simulink model "Battery_50kw_AC_500KW_400V_pruebas_2020_2_individual"  (R2020b)
settings: Solver=VariableStepAuto  StartTime=0.0  StopTime=0.4  RelTol=1e-3
InitFcn:
  | Ts=100e-6;
  | Timer=0.001;
StartFcn:
  | Ts=100e-6;
  | Timer=0.001;
undefined symbols (not defined in the file or in its folder): Ion, Lithium
libraries: powerlib x44, powerlib_meascontrol x16, slpidlib x10, simulink x5, electricdrivelib x1
(part 1 of 2)
settings Model: Creator=JGC  LastModifiedBy=DGY
settings DataIOCC: ReturnWorkspaceOutputs=off

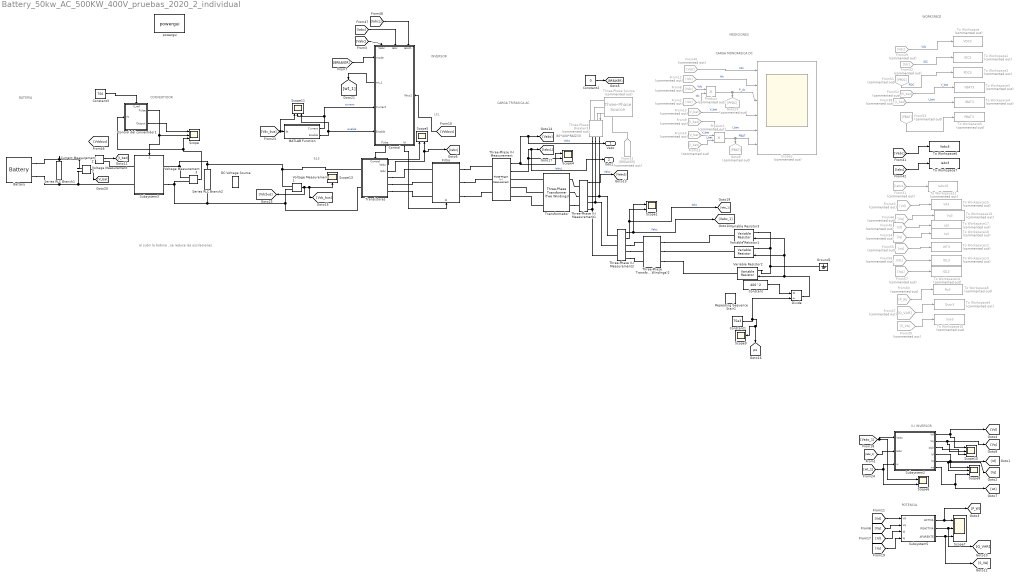
== system Battery_50kw_AC_500KW_400V_pruebas_2020_2_individual ==
  note: al subir la bobina , se reduce las oscilaciones
  note: WORKSPACE
  note: CARGA MONOFASICA DC
  note: MEDICIONES
  note: CONVERTIDOR
  note: INVERSOR
  note: BATERIA
  note: 80*400*RAIZ(3)
  note: CARGA TRIFASICA AC
  note: 615
  note: LCL
  note: V-I INVERSOR
  note: POTENCIA
  Battery : electricdrivelib/Extra Sources/Battery  BatType=Lithium-Ion  ShowTempParam=off  ThermalPreset=no  ShowAgeParam=off  NomV=512  NomQ=102400/512  SOC=70  Batt_Tr=30  PresetModel=on  MaxQ=200  MinV=384  FullV=595.9614  Dis_rate=86.9565  R=0.0256  Normal_OP=180.8696  expZone="[553.1576      9.826087]"  current=[6.5 13 32.5]  Units=Time  Tci=20  NomT=20  T2=-30  MaxQ2=4.8  FullV2=7.1  Normal_OP2=5.655  expZone2="[6.58           1]"  Rca=0.6  ti=2000  Dp=0  Neq0=0  Tsim=1e6  Ta1=25  Qeol=5.4*0.9  Reol=0.013333*1.2  Char_age=[2.3478, 3]  Dis_age=[2.3478, 10]  N1=1500  N2=10500  N3=1000  N4=1400  Ta2=45  N5=950
  Constant : Constant  Value=400^2
  Constant1 : Constant  Value=75e3
  Constant2 : Constant  Value=0
  Constant3 : Constant  Value=750
  "Control " : Subsystem
      settings: PortSchema="{\"entries\":[{\"content\":{\"sides\":[{\"content\":{\"connectorIds\":[\"In1\",\"Out3\",\"In2\",\"In3\"]},\"type\":\"ConnectorPlacement.EquallySpacedRectSide\",\"uuid\":\"040f479b-0063-4a97-945a-b7b76c14ccf9\"},{\"content\":{\"connectorIds\":[\"In7\"],\"side\":\"RIGHT\"},\"type\":\"ConnectorPlacement.EquallySpacedRectSide\",\"uuid\":\"48d15187-e0ba-47e4-acd1-e370322fb20d\"},{\"content\":{\"connectorIds\":[\"In4\",\"In5\",\"In6\"],\"side\":\"TOP\"},\"type\":\"ConnectorPlacement.EquallySpacedRectSide\",\"uuid\":\"c47ff363-741e-4c95-9660-92ffbbf0858a\"},{\"content\":{\"connectorIds\":[\"Out1\",\"Out2\"],\"side\":\"BOTTOM\"},\"type\":\"ConnectorPlacement.EquallySpacedRectSide\",\"uuid\":\"eb550659-5dfa-48af-9c5b-3062ad81491f\"}]},\"type\":\"ConnectorPlacement.EquallySpacedConnector\",\"uuid\":\"b4b94fd9-d3fa-4033-a0eb-720d35d74a7d\"}],\"packageUris\":[\"http://schema.mathworks.com/mf0/Connector/R2020b\"],\"version\":\"1.0\"}"
  Control del convertidor1 : Subsystem
      settings: PortSchema="{\"entries\":[{\"content\":{\"sides\":[{\"content\":{\"connectorIds\":[\"In1\"]},\"type\":\"ConnectorPlacement.EquallySpacedRectSide\",\"uuid\":\"952f4d9f-85a3-4809-ab80-f95b4e630059\"},{\"content\":{\"connectorIds\":[\"Out1\",\"Out2\"],\"side\":\"RIGHT\"},\"type\":\"ConnectorPlacement.EquallySpacedRectSide\",\"uuid\":\"24c0a236-3f22-4c40-86cc-925551a19bc9\"},{\"content\":{\"connectorIds\":[\"In2\"],\"side\":\"TOP\"},\"type\":\"ConnectorPlacement.EquallySpacedRectSide\",\"uuid\":\"1a366aec-943f-41ae-ba47-6c948c084703\"}]},\"type\":\"ConnectorPlacement.EquallySpacedConnector\",\"uuid\":\"c6d9e875-0dde-4ffd-9bd0-64114f723d5e\"}],\"packageUris\":[\"http://schema.mathworks.com/mf0/Connector/R2020b\"],\"version\":\"1.0\"}"
  Current Measurement2 : powerlib/Measurements/Current Measurement  PhasorSimulation=off  OutputType=Complex  PSBequivalent=0
  DC Voltage Source : powerlib/Electrical Sources/DC Voltage Source  Amplitude=750  Measurements=None
  Divide : Product  Inputs=*/
  Filtro : Subsystem
      settings: PortSchema="{\"entries\":[{\"content\":{\"sides\":[{\"content\":{\"connectorIds\":[\"LConn1\",\"LConn2\",\"LConn3\"]},\"type\":\"ConnectorPlacement.EquallySpacedRectSide\",\"uuid\":\"44f292cd-7929-4e59-9d40-ef793941fadf\"},{\"content\":{\"connectorIds\":[\"RConn1\",\"RConn2\",\"RConn3\"],\"side\":\"RIGHT\"},\"type\":\"ConnectorPlacement.EquallySpacedRectSide\",\"uuid\":\"e88b12c4-b753-4f44-a76b-0d232ef629de\"},{\"content\":{\"side\":\"TOP\"},\"type\":\"ConnectorPlacement.EquallySpacedRectSide\",\"uuid\":\"3a4dfe0a-8373-429f-aa79-480f87b68f50\"},{\"content\":{\"connectorIds\":[\"In1\"],\"side\":\"BOTTOM\"},\"type\":\"ConnectorPlacement.EquallySpacedRectSide\",\"uuid\":\"d1028483-6dfb-4af9-bac2-a2f24ebe33e6\"}]},\"type\":\"ConnectorPlacement.EquallySpacedConnector\",\"uuid\":\"17b3d09e-bad1-4b7f-8a8e-7737b1d04969\"}],\"packageUris\":[\"http://schema.mathworks.com/mf0/Connector/R2020b\"],\"version\":\"1.0\"}"
  From12 : From  Commented=on  GotoTag=Idc
  From13 : From  Commented=on  GotoTag=V_bat
  From14 : From  Commented=on  GotoTag=V_bat
  From15 : From  Commented=on  GotoTag=I_bat
  From2 : From  Commented=on  GotoTag=Idc
  From29 : From  Commented=on  GotoTag=Vdc
  From30 : From  Commented=on  GotoTag=P_W
  From31 : From  Commented=on  GotoTag=IabcL
  From32 : From  Commented=on  GotoTag=Idc
  From33 : From  Commented=on  GotoTag=BREAKER
  From37 : From  Commented=on  GotoTag=Q_VAR
  From38 : From  Commented=on  GotoTag=I_bat
  From39 : From  Commented=on  GotoTag=S_VA
  From40 : From  Commented=on  GotoTag=Vdc
  From43 : From  Commented=on  GotoTag=Vd
  From44 : From  Commented=on  GotoTag=Vq
  From45 : From  Commented=on  GotoTag=Id
  From51 : From  Commented=on  GotoTag=PPDC
  From52 : From  Commented=on  GotoTag=V_bat
  From53 : From  Commented=on  GotoTag=PBAT
  From54 : From  Commented=on  GotoTag=Iq
  From55 : From  Commented=on  GotoTag=wt
  From56 : From  Commented=on  GotoTag=IdL
  From57 : From  Commented=on  GotoTag=IqL
  From8 : From  Commented=on  GotoTag=Vdc
  From9 : From  Commented=on  GotoTag=I_bat
  Goto23 : Goto  Commented=on  GotoTag=PPDC
  Goto9 : Goto  Commented=on  GotoTag=PBAT
  Ground1 : powerlib/Elements/Ground  LConnTagsString=a
  MATLAB Function : MATLAB Function  TreatAsAtomicUnit=on
  Product : Product  Commented=on
  Product1 : Product  Commented=on
  Repeating Sequence Stair1 : simulink/Sources/Repeating Sequence Stair  OutValues=[ 30e3 35e3 45e3 50e3 40e3].'  tsamp=0.08  OutMin=[]  OutMax=[]  OutDataTypeStr=double  OutputDataTypeScalingMode=double  OutDataType=fixdt(0,8)  ConRadixGroup=Best Precision: Vector-wise  OutScaling=2^-12
  Scope{,7..8,10..11} (5 alike) : Scope  NumInputPorts=3
  Scope{1,4..6} (4 alike) : Scope  NumInputPorts=2
  Scope13 : Scope
  Scope2 : Scope  Commented=on  NumInputPorts=6
  Scope9 : Scope
  Series RLC Branch1 : powerlib/Elements/Series RLC Branch  LConnTagsString=__new0  RConnTagsString=__new0  BranchType=RC  Resistance=0.3  Inductance=1e-3  SetiL0=off  InitialCurrent=0  Capacitance=1e-6  Setx0=on  InitialVoltage=512  Measurements=None
  Series RLC Branch2 : powerlib/Elements/Series RLC Branch  LConnTagsString=__new0  RConnTagsString=__new0  BranchType=C  Resistance=0.2  Inductance=1e-3  SetiL0=off  InitialCurrent=0  Capacitance=0.15  Setx0=on  InitialVoltage=600  Measurements=None
  Subsystem2 : Subsystem
  Subsystem3 : Subsystem
      settings: PortSchema="{\"entries\":[{\"content\":{\"sides\":[{\"content\":{\"connectorIds\":[\"LConn1\",\"LConn2\"]},\"type\":\"ConnectorPlacement.EquallySpacedRectSide\",\"uuid\":\"7a980847-0fd3-4a52-ae22-59cd2a1ed559\"},{\"content\":{\"connectorIds\":[\"RConn1\",\"RConn2\"],\"side\":\"RIGHT\"},\"type\":\"ConnectorPlacement.EquallySpacedRectSide\",\"uuid\":\"85effeeb-73a6-4b0a-b51b-5eb0082317ff\"},{\"content\":{\"connectorIds\":[\"In1\"],\"side\":\"TOP\"},\"type\":\"ConnectorPlacement.EquallySpacedRectSide\",\"uuid\":\"eb55fae0-79ad-414f-ab96-49c332138803\"},{\"content\":{\"side\":\"BOTTOM\"},\"type\":\"ConnectorPlacement.EquallySpacedRectSide\",\"uuid\":\"1fd972ff-419a-4657-8ea4-57d89be2b868\"}]},\"type\":\"ConnectorPlacement.EquallySpacedConnector\",\"uuid\":\"1807473d-fd42-44e0-a7e4-668a7bf21429\"}],\"packageUris\":[\"http://schema.mathworks.com/mf0/Connector/R2020b\"],\"version\":\"1.0\"}"
  Subsystem5 : Subsystem
  Three-Phase Transformer (Two Windings)2 : powerlib/Elements/Three-Phase Transformer (Two Windings)  Winding1Connection=Yg  Winding2Connection=Yg  CoreType=Three single-phase transformers  SetSaturation=off  Hysteresis=off  DataFile='hysteresis'  SetInitialFlux=off  Measurements=None  UNITS=SI  NominalPower=[ 50e3 , 50 ]  Winding1=[400 0.0064 0]  Winding2=[400 0.0064 0]  Rm=1600  Lm=0  L0=0.5  Saturation=[0 0;0.24495 1.2475;102.06 1.5802]  InitialFluxes=[ 0.8 , -0.8 , 0.7 ]  BreakLoop=off  DiscreteSolver=Trapezoidal iterative  DataType=on  TransfoNumber=1
  Three-Phase V-I Measurement : powerlib/Measurements/Three-Phase V-I Measurement  VoltageMeasurement=phase-to-phase  SetLabelV=off  LabelV=Vabc  Vpu=off  VpuLL=off  CurrentMeasurement=yes  SetLabelI=off  LabelI=Iabc  Ipu=off  Pbase=100e6  Vbase=500e3  OutputType=Complex  PhasorSimulation=off  PSBequivalent=0
  Three-Phase V-I Measurement1 : powerlib/Measurements/Three-Phase V-I Measurement  VoltageMeasurement=phase-to-phase  SetLabelV=off  LabelV=Vabc  Vpu=off  VpuLL=off  CurrentMeasurement=yes  SetLabelI=off  LabelI=Iabc  Ipu=off  Pbase=100e6  Vbase=500e3  OutputType=Complex  PhasorSimulation=off  PSBequivalent=0
  Three-Phase V-I Measurement2 : powerlib/Measurements/Three-Phase V-I Measurement  VoltageMeasurement=phase-to-phase  SetLabelV=off  LabelV=Vabc  Vpu=off  VpuLL=off  CurrentMeasurement=yes  SetLabelI=off  LabelI=Iabc  Ipu=off  Pbase=100e6  Vbase=500e3  OutputType=Complex  PhasorSimulation=off  PSBequivalent=0
  Three-Phase Breaker3 : powerlib/Elements/Three-Phase Breaker  Commented=on  InitialState=closed  SwitchA=on  SwitchB=on  SwitchC=on  SwitchTimes="[1/60  5/60]"  External=on  BreakerResistance=0.01  SnubberResistance=1e6  SnubberCapacitance=inf  Measurements=None
  Three-Phase Source : powerlib/Electrical Sources/Three-Phase Source  Commented=on  InternalConnection=Y  VoltagePhases=off  Voltage=400  PhaseAngle=0  Voltage_phases=[25e3 25e3 25e3]/sqrt(3)  PhaseAngles_phases=[0 -120 +120]  Frequency=50  NonIdealSource=on  SpecifyImpedance=off  Resistance=0.0001e-3  Inductance=0.0001e-9  ShortCircuitLevel=100e6  BaseVoltage=400  XRratio=7  BusType=swing  Pref=10e3  Qref=0  Prefabc=[10e3, 10e3, 10e3]  Qrefabc=[0, 0, 0]  Qmin=-inf  Qmax=inf
  To Workspace : ToWorkspace  Commented=on  VariableName=VDC3  SaveFormat=Timeseries  SampleTime=-1
  To Workspace1 : ToWorkspace  Commented=on  VariableName=IDC3  SaveFormat=Timeseries  SampleTime=-1
  To Workspace10 : ToWorkspace  Commented=on  VariableName=Sva3  SaveFormat=Timeseries  SampleTime=-1
  To Workspace11 : ToWorkspace  Commented=on  VariableName=IabcL5  SaveFormat=Structure With Time  SampleTime=-1
  To Workspace12 : ToWorkspace  Commented=on  VariableName=WT3  SaveFormat=Timeseries  SampleTime=-1
  To Workspace13 : ToWorkspace  Commented=on  VariableName=IDL3  SaveFormat=Timeseries  SampleTime=-1
  To Workspace14 : ToWorkspace  Commented=on  VariableName=IQL3  SaveFormat=Timeseries  SampleTime=-1
  To Workspace15 : ToWorkspace  Commented=on  VariableName=Vd3  SaveFormat=Timeseries  SampleTime=-1
  To Workspace16 : ToWorkspace  Commented=on  VariableName=Vq3  SaveFormat=Timeseries  SampleTime=-1
  To Workspace17 : ToWorkspace  Commented=on  VariableName=Id3  SaveFormat=Timeseries  SampleTime=-1
  To Workspace18 : ToWorkspace  Commented=on  VariableName=Iq3  SaveFormat=Timeseries  SampleTime=-1
  To Workspace2 : ToWorkspace  Commented=on  VariableName=PDC3  SaveFormat=Timeseries  SampleTime=-1
  To Workspace3 : ToWorkspace  Commented=on  VariableName=VBAT3  SaveFormat=Timeseries  SampleTime=-1
  To Workspace4 : ToWorkspace  Commented=on  VariableName=IBAT3  SaveFormat=Timeseries  SampleTime=-1
  To Workspace5 : ToWorkspace  Commented=on  VariableName=PBAT3  SaveFormat=Timeseries  SampleTime=-1
  To Workspace6 : ToWorkspace  VariableName=Vabc5  SaveFormat=Structure With Time  SampleTime=-1
  To Workspace7 : ToWorkspace  VariableName=Iabc3  SaveFormat=Timeseries  SampleTime=-1
  To Workspace8 : ToWorkspace  Commented=on  VariableName=Pw3  SaveFormat=Timeseries  SampleTime=-1
  To Workspace9 : ToWorkspace  Commented=on  VariableName=Qvar3  SaveFormat=Timeseries  SampleTime=-1
  "Transformador " : powerlib/Elements/Three-Phase Transformer (Two Windings)  Winding1Connection=Yg  Winding2Connection=Yg  CoreType=Three single-phase transformers  SetSaturation=off  Hysteresis=off  DataFile='hysteresis'  SetInitialFlux=off  Measurements=None  UNITS=SI  NominalPower=[50e3 , 50 ]  Winding1=[400 0.0064 0]  Winding2=[400 0.0064 0]  Rm=1600  Lm=0  L0=0.5  Saturation=[0 0;0.24495 1.2475;102.06 1.5802]  InitialFluxes=[ 0.8 , -0.8 , 0.7 ]  BreakLoop=off  DiscreteSolver=Trapezoidal iterative  DataType=on  TransfoNumber=1
  Transistores : Subsystem
      settings: PortSchema="{\"entries\":[{\"content\":{\"sides\":[{\"content\":{\"connectorIds\":[\"LConn1\",\"LConn2\"]},\"type\":\"ConnectorPlacement.EquallySpacedRectSide\",\"uuid\":\"4b4a90af-a54c-4879-a767-640ef5f3fcb3\"},{\"content\":{\"connectorIds\":[\"Out1\",\"Out2\",\"RConn1\",\"RConn2\",\"RConn3\"],\"side\":\"RIGHT\"},\"type\":\"ConnectorPlacement.EquallySpacedRectSide\",\"uuid\":\"9175716d-9f9b-4229-800b-ed18d0bc4919\"},{\"content\":{\"connectorIds\":[\"In1\"],\"side\":\"TOP\"},\"type\":\"ConnectorPlacement.EquallySpacedRectSide\",\"uuid\":\"ad8bb3e4-0cf0-4c72-aeb3-553776322e14\"}]},\"type\":\"ConnectorPlacement.EquallySpacedConnector\",\"uuid\":\"7a2ee168-b262-4afb-be64-1e845efa873f\"}],\"packageUris\":[\"http://schema.mathworks.com/mf0/Connector/R2020b\"],\"version\":\"1.0\"}"
  Variable Resistor1 : powerlib/Elements/Variable Resistor  Rabsmin=1e-3
      settings: SourceProductBaseCode=PS
  Variable Resistor2 : powerlib/Elements/Variable Resistor  Rabsmin=1e-3
      settings: SourceProductBaseCode=PS
  Variable Resistor3 : powerlib/Elements/Variable Resistor  Rabsmin=1e-3
      settings: SourceProductBaseCode=PS
  Voltage Measurement1 : powerlib/Measurements/Voltage Measurement  PhasorSimulation=off  OutputType=Complex  PSBequivalent=0
  Voltage Measurement2 : powerlib/Measurements/Voltage Measurement  PhasorSimulation=off  OutputType=Complex  PSBequivalent=0
  Voltage Measurement3 : powerlib/Measurements/Voltage Measurement  PhasorSimulation=off  OutputType=Complex  PSBequivalent=0
  powergui : powerlib/powergui  Priority=1  SimulationMode=Discrete  SampleTime=1e-5*3  frequency=60  Iterations=50  frequencyindice=0  Pbase=100e6  ErrMax=1e-4  UnitsV=kV  UnitsW=MW  buscounter=0  FunctionMessages=off  echomessages=off  EnableUseOfTLC=off  CurrentSourceSwitches=off  DisableSnubberDevices=off  DisableRonSwitches=off  DisableVfSwitches=off  DisplayEquations=off  AutomaticDiscreteSolvers=off  SolverType=Tustin/Backward Euler (TBE)  Interpol=off  ExternalGateDelay=off  methode=off  Ts=100  x0status=blocks  SPID=on  SwTol=0  HookPort=off  NonlinearTolerance=1e-4  nMaxIteration=100  ContinueOnMaxIteration=off  RestoreLinks=warning  ResistiveCurrentMeasurement=off  Frange=[0:2:500]  Ylog=off  Xlog=on  ShowGrid=off  save=off  variable=ZData  structure=IDC  ZoomFFT=off  StartTime=0.01  cycles=7  DisplayStyle=1  fundamental=50  FreqAxis=off  MaxFrequency=10000  frequencyindicesteady=1  RmsSteady=1  display=off
  Vabc : Outport
  IabcL : Outport  Port=2
  tag scope: po=global
  wires:
  MATLAB Function/1(Current) -> Scope11/2, "Control "/2(Current)  "current"
  [BREAKER] -> "Control "/1(mode)
  From32/1 -> To Workspace1/1  "IDC"
  From30/1 -> To Workspace8/1
  From38/1 -> To Workspace4/1  "I_bat"
  From29/1 -> To Workspace/1  "Vdc"
  From45/1 -> To Workspace17/1
  [Vdc_bus] -> MATLAB Function/1(IN), Scope11/1
  From37/1 -> To Workspace9/1
  Transistores/1(Vabc) -> Scope5/1
  [Vdcbus] -> "Control "/7(Vbus1)
  From57/1 -> To Workspace14/1
  From51/1 -> To Workspace2/1  "PDC"
  From2/1 -> Product/2  "Idc"
  [Iabc] -> To Workspace7/1
  From52/1 -> To Workspace3/1  "V_bat"
  From39/1 -> To Workspace10/1
  From53/1 -> To Workspace5/1
  From54/1 -> To Workspace18/1
  From56/1 -> To Workspace13/1
  From40/1 -> Scope2/1  "Vdc"
  From44/1 -> To Workspace16/1
  Transistores/2(Iabc) -> Scope5/2, [Iabc]
  Product1/1 -> Goto9/1, Scope2/6  "PBAT"
  From9/1 -> Scope2/5  "I_bat"
  Product/1 -> Goto23/1, Scope2/3  "P_dc"
  From8/1 -> Product/1  "Vdc"
  From13/1 -> Scope2/4  "V_bat"
  From14/1 -> Product1/1  "V_bat"
  From12/1 -> Scope2/2  "Idc"
  "Control "/1(Pulse) -> Transistores/1(Control)
  From15/1 -> Product1/2  "I_bat"
  From31/1 -> To Workspace11/1
  [Vabc] -> To Workspace6/1
  From55/1 -> To Workspace12/1
  Three-Phase V-I Measurement/1 -> Scope4/1, [Vabc], Vabc/1  "Vabc"
  From43/1 -> To Workspace15/1
  Three-Phase V-I Measurement/2 -> Scope4/2, [IabcL], IabcL/1  "IabcL"
  MATLAB Function/2(Enable) -> Scope11/3, "Control "/3(Enable)  "enable"
  Divide/1 -> Variable Resistor2/1, Variable Resistor3/1, Variable Resistor1/1
  Constant/1 -> Divide/1
  Three-Phase V-I Measurement1/1 -> [VabcS]  "Vabc"
  Constant2/1 -> [BREAKER]
  From33/1 -> Three-Phase Breaker3/1
  Voltage Measurement1/1 -> [Vdcbus], Scope13/1, [Vdc_bus]
  "Control "/2(Id) -> Filtro/1(Id)
  Control del convertidor1/1(Pulse) -> Subsystem3/1(S), Scope/2
  Voltage Measurement2/1 -> [V_bat]
  Current Measurement2/1 -> [I_bat]
  Voltage Measurement3/1 -> Control del convertidor1/1(Vs), Scope/3
  Constant3/1 -> Control del convertidor1/2(V_ref)
  Control del convertidor1/2(Output) -> Scope/1
  Constant1/1 -> Divide/2, Scope9/1, [po]
  [Vabc] -> "Control "/4(Vabc)
  [Iabc] -> "Control "/5(Iabc)
  [IabcL] -> "Control "/6(Iabcl1)
  Three-Phase V-I Measurement2/1 -> [Vabc_1], Scope1/1  "Vabc"
  Three-Phase V-I Measurement2/2 -> [Iabc_1], Scope1/2  "Iabc"
  Subsystem2/2(Vq) -> Scope10/2, [Vq]
  [Id] -> Subsystem5/3(Id)
  Subsystem5/1(ACTIVA) -> [P_W], Scope7/1
  Subsystem2/1(Vd) -> Scope10/1, [Vd]
  [Iq] -> Subsystem5/4(Iq)
  [Vabc_1] -> Scope6/1, Subsystem2/1(Vabc)
  Subsystem5/3(APARENTE) -> [S_VA], Scope7/3
  [Vd] -> Subsystem5/1(Vd)
  [Iabc_1] -> Subsystem2/2(Iabc)
  [Vq] -> Subsystem5/2(Vq)
  Subsystem2/3(dq0) -> Scope10/3
  [wt_1] -> Subsystem2/3(w), Scope6/2
  Subsystem2/6(wt) -> [wt], Scope8/3
  Subsystem2/4(Id) -> [Id], Scope8/1
  Subsystem5/2(REACTIVA) -> [Q_VAR], Scope7/2
  Subsystem2/5(Iq) -> Scope8/2, [Iq]
  "Control "/3(wt_1) -> [wt_1]
  connections:
  Filtro/LConn3 -- Three-Phase V-I Measurement/LConn3
  Transistores/RConn1 -- Filtro/RConn1
  Transistores/RConn2 -- Filtro/RConn2
  Filtro/LConn1 -- Three-Phase V-I Measurement/LConn1
  Filtro/LConn2 -- Three-Phase V-I Measurement/LConn2
  Transistores/RConn3 -- Filtro/RConn3
  Variable Resistor3/LConn1 -- Variable Resistor1/LConn1 -- Variable Resistor2/LConn1 -- Ground1/LConn1
  Three-Phase V-I Measurement1/RConn1 -- Three-Phase Breaker3/RConn1 -- Three-Phase V-I Measurement2/LConn1
  Three-Phase V-I Measurement1/RConn2 -- Three-Phase Breaker3/RConn2 -- Three-Phase V-I Measurement2/LConn2
  Three-Phase V-I Measurement1/RConn3 -- Three-Phase Breaker3/RConn3 -- Three-Phase V-I Measurement2/LConn3
  "Transformador "/LConn2 -- Three-Phase V-I Measurement/RConn2
  "Transformador "/LConn3 -- Three-Phase V-I Measurement/RConn3
  Three-Phase V-I Measurement1/LConn1 -- "Transformador "/RConn1
  "Transformador "/RConn2 -- Three-Phase V-I Measurement1/LConn2
  "Transformador "/LConn1 -- Three-Phase V-I Measurement/RConn1
  "Transformador "/RConn3 -- Three-Phase V-I Measurement1/LConn3
  Three-Phase Source/RConn2 -- Three-Phase Breaker3/LConn2
  Three-Phase Source/RConn1 -- Three-Phase Breaker3/LConn1
  Three-Phase Source/RConn3 -- Three-Phase Breaker3/LConn3
  Series RLC Branch1/LConn1 -- Battery/LConn1 -- Voltage Measurement2/LConn1 -- Current Measurement2/LConn1
  Series RLC Branch1/RConn1 -- Battery/LConn2 -- Voltage Measurement2/LConn2 -- Subsystem3/LConn2
  Subsystem3/LConn1 -- Current Measurement2/RConn1
  Subsystem3/RConn2 -- Voltage Measurement3/LConn2 -- Transistores/LConn2 -- Voltage Measurement1/LConn2 -- Series RLC Branch2/RConn1
  Subsystem3/RConn1 -- Voltage Measurement1/LConn1 -- Transistores/LConn1 -- Series RLC Branch2/LConn1 -- Voltage Measurement3/LConn1
  Three-Phase V-I Measurement2/RConn1 -- Three-Phase Transformer (Two Windings)2/LConn1
  Three-Phase V-I Measurement2/RConn2 -- Three-Phase Transformer (Two Windings)2/LConn2
  Three-Phase V-I Measurement2/RConn3 -- Three-Phase Transformer (Two Windings)2/LConn3
  Three-Phase Transformer (Two Windings)2/RConn1 -- Variable Resistor3/RConn1
  Three-Phase Transformer (Two Windings)2/RConn2 -- Variable Resistor1/RConn1
  Three-Phase Transformer (Two Windings)2/RConn3 -- Variable Resistor2/RConn1

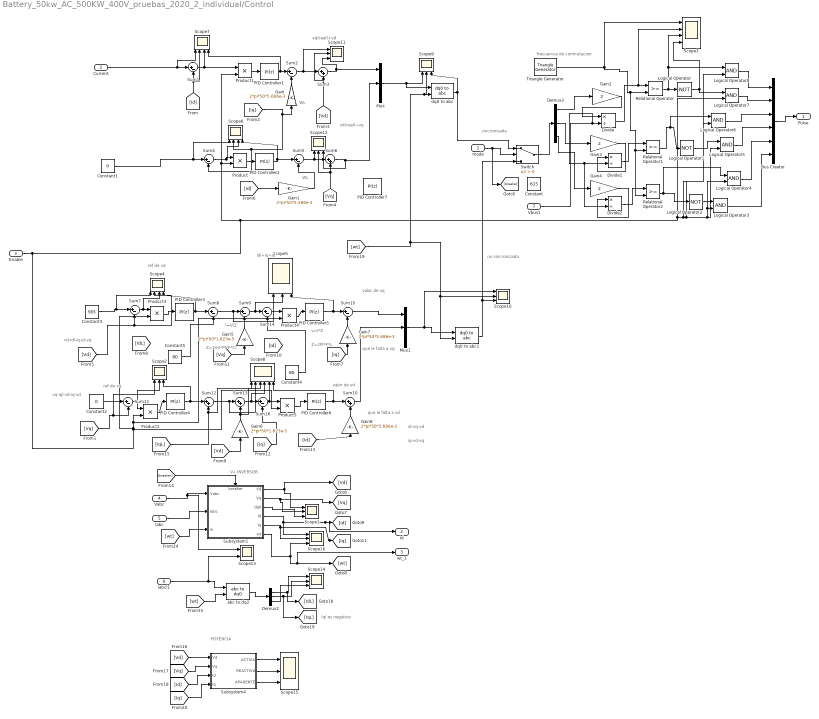
== system Battery_50kw_AC_500KW_400V_pruebas_2020_2_individual/Control  ==
  note: v=I*Z
  note: Z=2PI*F*L
  note: vd-idl-iq-id-vq
  note: ref de vq
  note: que le falta a vd
  note: ref de vd
  note: que le falta a vq
  note: valor de vq
  note: iq-vd-vq
  note: valor de vd
  note: vq-iql-vd-iq-vd
  note: I=V/Z
  note: Z=1/(2*PI*F*C)
  note: id-vq-vd
  note: idl+iq+id
  note: vq(real)+vd
  note: vd(real)+vq
  note: WL
  note: WL
  note: frecuencia de conmutacion
  note: no sincronizada
  note: sincronizada
  note: POTENCIA
  note: V-I INVERSOR
  note: Iql es negativo
  mode : Inport
  Current : Inport  Port=2
  Enable : Inport  Port=3
  Vabc : Inport  Port=4
  Iabc : Inport  Port=5
  Iabcl1 : Inport  Port=6
  Vbus1 : Inport  Port=7
  Bus Creator : BusCreator  Inputs=6
  Constant : Constant  Value=615
  Constant1 : Constant  Value=0
  Constant2 : Constant  Value=0
  Constant3 : Constant  Value=565
  Constant4 : Constant  Value=80
  Constant5 : Constant  Value=80
  Demux2 : Demux  Outputs=3
  Demux3 : Demux  Outputs=3
  Divide : Product  Inputs=*/
  Divide1 : Product  Inputs=*/
  Divide2 : Product  Inputs=*/
  Gain : Gain  Gain=2*pi*50*5.686e-3
  Gain1 : Gain  Gain=2*pi*50*5.586e-3
  Gain2 : Gain  Gain=2
  Gain3 : Gain  Gain=2
  Gain4 : Gain  Gain=2
  Gain5 : Gain  Gain=2*pi*50*1.823e-5
  Gain6 : Gain  Gain=2*pi*50*1.823e-5
  Gain7 : Gain  Gain=2*pi*50*5.686e-3
  Gain8 : Gain  Gain=2*pi*50*5.686e-3
  Logical Operator : Logic  Operator=NOT  AllPortsSameDT=off  OutDataTypeStr=boolean
  Logical Operator1 : Logic  Operator=NOT  AllPortsSameDT=off  OutDataTypeStr=boolean
  Logical Operator2 : Logic  Operator=NOT  AllPortsSameDT=off  OutDataTypeStr=boolean
  Logical Operator{3..8} (6 alike) : Logic  AllPortsSameDT=off  OutDataTypeStr=boolean
  Mux : Mux  Inputs=3
  Mux1 : Mux  Inputs=3
  PID Controller1 : slpidlib/PID Controller  Controller=PI  Form=Parallel  TimeDomain=Discrete-time  UseExternalTs=off  SampleTime=Ts  IntegratorMethod=Forward Euler  FilterMethod=Forward Euler  ControllerParametersSource=internal  P=60  I=0  D=0  UseFilter=on  N=100  TunerSelectOption=Transfer Function Based (PID Tuner App)  InitialConditionSource=internal  InitialConditionForIntegrator=0  InitialConditionForFilter=0  DifferentiatorICPrevScaledInput=0  ExternalReset=none  TrackingMode=off  Kt=1  LimitOutput=off  SatLimitsSource=internal  UpperSaturationLimit=inf  LowerSaturationLimit=-inf  LinearizeAsGain=on  AntiWindupMode=none  Kb=1  POutMin=[]  POutMax=[]  IOutMin=[]  IOutMax=[]  DOutMin=[]  DOutMax=[]  NOutMin=[]  NOutMax=[]  SumOutMin=[]  SumOutMax=[]  SaturationOutMin=[]  SaturationOutMax=[]  PParamMin=[]  PParamMax=[]  IParamMin=[]  IParamMax=[]  DParamMin=[]  DParamMax=[]  NParamMin=[]  NParamMax=[]  KbParamMin=[]  KbParamMax=[]  KtParamMin=[]  KtParamMax=[]  KbOutMin=[]  KbOutMax=[]  KtOutMin=[]  KtOutMax=[]  IntegratorOutMin=[]  IntegratorOutMax=[]  FilterOutMin=[]  FilterOutMax=[]  SumI1OutMin=[]  SumI1OutMax=[]  SumI2OutMin=[]  SumI2OutMax=[]  SumI3OutMin=[]  SumI3OutMax=[]  SumI4OutMin=[]  SumI4OutMax=[]  SumDOutMin=[]  SumDOutMax=[]  DifferentiatorOutMin=[]  DifferentiatorOutMax=[]  FilterDiffOutCoefMin=[]  FilterDiffOutCoefMax=[]  ReciprocalOutMin=[]  ReciprocalOutMax=[]  SumDenOutMin=[]  SumDenOutMax=[]  SumNumOutMin=[]  SumNumOutMax=[]  DivideOutMin=[]  DivideOutMax=[]  UdiffTsProdOutMin=[]  UdiffTsProdOutMax=[]  NTsProdOutMin=[]  NTsProdOutMax=[]  UintegralTsProdOutMin=[]  UintegralTsProdOutMax=[]  UngainTsProdOutMin=[]  UngainTsProdOutMax=[]  IntegratorContinuousStateAttributes=''  IntegratorStateMustResolveToSignalObject=off  IntegratorRTWStateStorageClass=Auto  FilterContinuousStateAttributes=''  FilterStateMustResolveToSignalObject=off  FilterRTWStateStorageClass=Auto  ParallelPVariant=InternalParameters  IdealPVariant=Disabled  IVariant=InternalParameters  DVariant=Disabled  IntegratorVariant=Discrete  SatVariant=Disabled  AWVariant=Passthrough  PCopyVariant=Disabled  TRVariant=Disabled  FdbkBlocksVariant=Forward  IdealPFdbkVariant=Disabled  SatFdbkVariant=Disabled  DerivativeFilterVariant=Disabled  NVariant=Disabled  NCopyVariant=Disabled_SignalSpec  FilterICVariant=Disabled  IntegratorICVariant=InternalICs  ExternalResetVariant=Disabled  TRSumVariant=Passthrough  SumFdbkVariant=Disabled  SumVariant=Sum_PI  TsampFilterVariant=InternalTs  TsampNgainVariant=Passthrough  TsampIntegralVariant=Passthrough  ExternalSaturationOutDataTypeStr=Inherit: Same as second input
  PID Controller2 : slpidlib/PID Controller  Controller=PI  Form=Parallel  TimeDomain=Discrete-time  UseExternalTs=off  SampleTime=Ts  IntegratorMethod=Forward Euler  FilterMethod=Forward Euler  ControllerParametersSource=internal  P=70  I=10  D=0  UseFilter=on  N=100  TunerSelectOption=Transfer Function Based (PID Tuner App)  InitialConditionSource=internal  InitialConditionForIntegrator=0  InitialConditionForFilter=0  DifferentiatorICPrevScaledInput=0  ExternalReset=none  TrackingMode=off  Kt=1  LimitOutput=off  SatLimitsSource=internal  UpperSaturationLimit=inf  LowerSaturationLimit=-inf  LinearizeAsGain=on  AntiWindupMode=none  Kb=1  POutMin=[]  POutMax=[]  IOutMin=[]  IOutMax=[]  DOutMin=[]  DOutMax=[]  NOutMin=[]  NOutMax=[]  SumOutMin=[]  SumOutMax=[]  SaturationOutMin=[]  SaturationOutMax=[]  PParamMin=[]  PParamMax=[]  IParamMin=[]  IParamMax=[]  DParamMin=[]  DParamMax=[]  NParamMin=[]  NParamMax=[]  KbParamMin=[]  KbParamMax=[]  KtParamMin=[]  KtParamMax=[]  KbOutMin=[]  KbOutMax=[]  KtOutMin=[]  KtOutMax=[]  IntegratorOutMin=[]  IntegratorOutMax=[]  FilterOutMin=[]  FilterOutMax=[]  SumI1OutMin=[]  SumI1OutMax=[]  SumI2OutMin=[]  SumI2OutMax=[]  SumI3OutMin=[]  SumI3OutMax=[]  SumI4OutMin=[]  SumI4OutMax=[]  SumDOutMin=[]  SumDOutMax=[]  DifferentiatorOutMin=[]  DifferentiatorOutMax=[]  FilterDiffOutCoefMin=[]  FilterDiffOutCoefMax=[]  ReciprocalOutMin=[]  ReciprocalOutMax=[]  SumDenOutMin=[]  SumDenOutMax=[]  SumNumOutMin=[]  SumNumOutMax=[]  DivideOutMin=[]  DivideOutMax=[]  UdiffTsProdOutMin=[]  UdiffTsProdOutMax=[]  NTsProdOutMin=[]  NTsProdOutMax=[]  UintegralTsProdOutMin=[]  UintegralTsProdOutMax=[]  UngainTsProdOutMin=[]  UngainTsProdOutMax=[]  IntegratorContinuousStateAttributes=''  IntegratorStateMustResolveToSignalObject=off  IntegratorRTWStateStorageClass=Auto  FilterContinuousStateAttributes=''  FilterStateMustResolveToSignalObject=off  FilterRTWStateStorageClass=Auto  ParallelPVariant=InternalParameters  IdealPVariant=Disabled  IVariant=InternalParameters  DVariant=Disabled  IntegratorVariant=Discrete  SatVariant=Disabled  AWVariant=Passthrough  PCopyVariant=Disabled  TRVariant=Disabled  FdbkBlocksVariant=Forward  IdealPFdbkVariant=Disabled  SatFdbkVariant=Disabled  DerivativeFilterVariant=Disabled  NVariant=Disabled  NCopyVariant=Disabled_SignalSpec  FilterICVariant=Disabled  IntegratorICVariant=InternalICs  ExternalResetVariant=Disabled  TRSumVariant=Passthrough  SumFdbkVariant=Disabled  SumVariant=Sum_PI  TsampFilterVariant=InternalTs  TsampNgainVariant=Passthrough  TsampIntegralVariant=Passthrough  ExternalSaturationOutDataTypeStr=Inherit: Same as second input
  PID Controller3 : slpidlib/PID Controller  Controller=PI  Form=Parallel  TimeDomain=Discrete-time  UseExternalTs=off  SampleTime=Ts  IntegratorMethod=Forward Euler  FilterMethod=Forward Euler  ControllerParametersSource=internal  P=1  I=80  D=0  UseFilter=on  N=100  TunerSelectOption=Transfer Function Based (PID Tuner App)  InitialConditionSource=internal  InitialConditionForIntegrator=0  InitialConditionForFilter=0  DifferentiatorICPrevScaledInput=0  ExternalReset=none  TrackingMode=off  Kt=1  LimitOutput=off  SatLimitsSource=internal  UpperSaturationLimit=inf  LowerSaturationLimit=-inf  LinearizeAsGain=on  AntiWindupMode=none  Kb=1  POutMin=[]  POutMax=[]  IOutMin=[]  IOutMax=[]  DOutMin=[]  DOutMax=[]  NOutMin=[]  NOutMax=[]  SumOutMin=[]  SumOutMax=[]  SaturationOutMin=[]  SaturationOutMax=[]  PParamMin=[]  PParamMax=[]  IParamMin=[]  IParamMax=[]  DParamMin=[]  DParamMax=[]  NParamMin=[]  NParamMax=[]  KbParamMin=[]  KbParamMax=[]  KtParamMin=[]  KtParamMax=[]  KbOutMin=[]  KbOutMax=[]  KtOutMin=[]  KtOutMax=[]  IntegratorOutMin=[]  IntegratorOutMax=[]  FilterOutMin=[]  FilterOutMax=[]  SumI1OutMin=[]  SumI1OutMax=[]  SumI2OutMin=[]  SumI2OutMax=[]  SumI3OutMin=[]  SumI3OutMax=[]  SumI4OutMin=[]  SumI4OutMax=[]  SumDOutMin=[]  SumDOutMax=[]  DifferentiatorOutMin=[]  DifferentiatorOutMax=[]  FilterDiffOutCoefMin=[]  FilterDiffOutCoefMax=[]  ReciprocalOutMin=[]  ReciprocalOutMax=[]  SumDenOutMin=[]  SumDenOutMax=[]  SumNumOutMin=[]  SumNumOutMax=[]  DivideOutMin=[]  DivideOutMax=[]  UdiffTsProdOutMin=[]  UdiffTsProdOutMax=[]  NTsProdOutMin=[]  NTsProdOutMax=[]  UintegralTsProdOutMin=[]  UintegralTsProdOutMax=[]  UngainTsProdOutMin=[]  UngainTsProdOutMax=[]  IntegratorContinuousStateAttributes=''  IntegratorStateMustResolveToSignalObject=off  IntegratorRTWStateStorageClass=Auto  FilterContinuousStateAttributes=''  FilterStateMustResolveToSignalObject=off  FilterRTWStateStorageClass=Auto  ParallelPVariant=InternalParameters  IdealPVariant=Disabled  IVariant=InternalParameters  DVariant=Disabled  IntegratorVariant=Discrete  SatVariant=Disabled  AWVariant=Passthrough  PCopyVariant=Disabled  TRVariant=Disabled  FdbkBlocksVariant=Forward  IdealPFdbkVariant=Disabled  SatFdbkVariant=Disabled  DerivativeFilterVariant=Disabled  NVariant=Disabled  NCopyVariant=Disabled_SignalSpec  FilterICVariant=Disabled  IntegratorICVariant=InternalICs  ExternalResetVariant=Disabled  TRSumVariant=Passthrough  SumFdbkVariant=Disabled  SumVariant=Sum_PI  TsampFilterVariant=InternalTs  TsampNgainVariant=Passthrough  TsampIntegralVariant=Passthrough  ExternalSaturationOutDataTypeStr=Inherit: Same as second input
  PID Controller4 : slpidlib/PID Controller  Controller=PI  Form=Parallel  TimeDomain=Discrete-time  UseExternalTs=off  SampleTime=Ts  IntegratorMethod=Forward Euler  FilterMethod=Forward Euler  ControllerParametersSource=internal  P=0.1  I=30  D=0  UseFilter=on  N=100  TunerSelectOption=Transfer Function Based (PID Tuner App)  InitialConditionSource=internal  InitialConditionForIntegrator=0  InitialConditionForFilter=0  DifferentiatorICPrevScaledInput=0  ExternalReset=none  TrackingMode=off  Kt=1  LimitOutput=off  SatLimitsSource=internal  UpperSaturationLimit=inf  LowerSaturationLimit=-inf  LinearizeAsGain=on  AntiWindupMode=none  Kb=1  POutMin=[]  POutMax=[]  IOutMin=[]  IOutMax=[]  DOutMin=[]  DOutMax=[]  NOutMin=[]  NOutMax=[]  SumOutMin=[]  SumOutMax=[]  SaturationOutMin=[]  SaturationOutMax=[]  PParamMin=[]  PParamMax=[]  IParamMin=[]  IParamMax=[]  DParamMin=[]  DParamMax=[]  NParamMin=[]  NParamMax=[]  KbParamMin=[]  KbParamMax=[]  KtParamMin=[]  KtParamMax=[]  KbOutMin=[]  KbOutMax=[]  KtOutMin=[]  KtOutMax=[]  IntegratorOutMin=[]  IntegratorOutMax=[]  FilterOutMin=[]  FilterOutMax=[]  SumI1OutMin=[]  SumI1OutMax=[]  SumI2OutMin=[]  SumI2OutMax=[]  SumI3OutMin=[]  SumI3OutMax=[]  SumI4OutMin=[]  SumI4OutMax=[]  SumDOutMin=[]  SumDOutMax=[]  DifferentiatorOutMin=[]  DifferentiatorOutMax=[]  FilterDiffOutCoefMin=[]  FilterDiffOutCoefMax=[]  ReciprocalOutMin=[]  ReciprocalOutMax=[]  SumDenOutMin=[]  SumDenOutMax=[]  SumNumOutMin=[]  SumNumOutMax=[]  DivideOutMin=[]  DivideOutMax=[]  UdiffTsProdOutMin=[]  UdiffTsProdOutMax=[]  NTsProdOutMin=[]  NTsProdOutMax=[]  UintegralTsProdOutMin=[]  UintegralTsProdOutMax=[]  UngainTsProdOutMin=[]  UngainTsProdOutMax=[]  IntegratorContinuousStateAttributes=''  IntegratorStateMustResolveToSignalObject=off  IntegratorRTWStateStorageClass=Auto  FilterContinuousStateAttributes=''  FilterStateMustResolveToSignalObject=off  FilterRTWStateStorageClass=Auto  ParallelPVariant=InternalParameters  IdealPVariant=Disabled  IVariant=InternalParameters  DVariant=Disabled  IntegratorVariant=Discrete  SatVariant=Disabled  AWVariant=Passthrough  PCopyVariant=Disabled  TRVariant=Disabled  FdbkBlocksVariant=Forward  IdealPFdbkVariant=Disabled  SatFdbkVariant=Disabled  DerivativeFilterVariant=Disabled  NVariant=Disabled  NCopyVariant=Disabled_SignalSpec  FilterICVariant=Disabled  IntegratorICVariant=InternalICs  ExternalResetVariant=Disabled  TRSumVariant=Passthrough  SumFdbkVariant=Disabled  SumVariant=Sum_PI  TsampFilterVariant=InternalTs  TsampNgainVariant=Passthrough  TsampIntegralVariant=Passthrough  ExternalSaturationOutDataTypeStr=Inherit: Same as second input
  PID Controller5 : slpidlib/PID Controller  Controller=PI  Form=Parallel  TimeDomain=Discrete-time  UseExternalTs=off  SampleTime=Ts  IntegratorMethod=Forward Euler  FilterMethod=Forward Euler  ControllerParametersSource=internal  P=10  I=30  D=0  UseFilter=on  N=100  TunerSelectOption=Transfer Function Based (PID Tuner App)  InitialConditionSource=internal  InitialConditionForIntegrator=0  InitialConditionForFilter=0  DifferentiatorICPrevScaledInput=0  ExternalReset=none  TrackingMode=off  Kt=1  LimitOutput=off  SatLimitsSource=internal  UpperSaturationLimit=inf  LowerSaturationLimit=-inf  LinearizeAsGain=on  AntiWindupMode=none  Kb=1  POutMin=[]  POutMax=[]  IOutMin=[]  IOutMax=[]  DOutMin=[]  DOutMax=[]  NOutMin=[]  NOutMax=[]  SumOutMin=[]  SumOutMax=[]  SaturationOutMin=[]  SaturationOutMax=[]  PParamMin=[]  PParamMax=[]  IParamMin=[]  IParamMax=[]  DParamMin=[]  DParamMax=[]  NParamMin=[]  NParamMax=[]  KbParamMin=[]  KbParamMax=[]  KtParamMin=[]  KtParamMax=[]  KbOutMin=[]  KbOutMax=[]  KtOutMin=[]  KtOutMax=[]  IntegratorOutMin=[]  IntegratorOutMax=[]  FilterOutMin=[]  FilterOutMax=[]  SumI1OutMin=[]  SumI1OutMax=[]  SumI2OutMin=[]  SumI2OutMax=[]  SumI3OutMin=[]  SumI3OutMax=[]  SumI4OutMin=[]  SumI4OutMax=[]  SumDOutMin=[]  SumDOutMax=[]  DifferentiatorOutMin=[]  DifferentiatorOutMax=[]  FilterDiffOutCoefMin=[]  FilterDiffOutCoefMax=[]  ReciprocalOutMin=[]  ReciprocalOutMax=[]  SumDenOutMin=[]  SumDenOutMax=[]  SumNumOutMin=[]  SumNumOutMax=[]  DivideOutMin=[]  DivideOutMax=[]  UdiffTsProdOutMin=[]  UdiffTsProdOutMax=[]  NTsProdOutMin=[]  NTsProdOutMax=[]  UintegralTsProdOutMin=[]  UintegralTsProdOutMax=[]  UngainTsProdOutMin=[]  UngainTsProdOutMax=[]  IntegratorContinuousStateAttributes=''  IntegratorStateMustResolveToSignalObject=off  IntegratorRTWStateStorageClass=Auto  FilterContinuousStateAttributes=''  FilterStateMustResolveToSignalObject=off  FilterRTWStateStorageClass=Auto  ParallelPVariant=InternalParameters  IdealPVariant=Disabled  IVariant=InternalParameters  DVariant=Disabled  IntegratorVariant=Discrete  SatVariant=Disabled  AWVariant=Passthrough  PCopyVariant=Disabled  TRVariant=Disabled  FdbkBlocksVariant=Forward  IdealPFdbkVariant=Disabled  SatFdbkVariant=Disabled  DerivativeFilterVariant=Disabled  NVariant=Disabled  NCopyVariant=Disabled_SignalSpec  FilterICVariant=Disabled  IntegratorICVariant=InternalICs  ExternalResetVariant=Disabled  TRSumVariant=Passthrough  SumFdbkVariant=Disabled  SumVariant=Sum_PI  TsampFilterVariant=InternalTs  TsampNgainVariant=Passthrough  TsampIntegralVariant=Passthrough  ExternalSaturationOutDataTypeStr=Inherit: Same as second input
  PID Controller6 : slpidlib/PID Controller  Controller=PI  Form=Parallel  TimeDomain=Discrete-time  UseExternalTs=off  SampleTime=Ts  IntegratorMethod=Forward Euler  FilterMethod=Forward Euler  ControllerParametersSource=internal  P=10  I=30  D=0  UseFilter=on  N=100  TunerSelectOption=Transfer Function Based (PID Tuner App)  InitialConditionSource=internal  InitialConditionForIntegrator=0  InitialConditionForFilter=0  DifferentiatorICPrevScaledInput=0  ExternalReset=none  TrackingMode=off  Kt=1  LimitOutput=off  SatLimitsSource=internal  UpperSaturationLimit=inf  LowerSaturationLimit=-inf  LinearizeAsGain=on  AntiWindupMode=none  Kb=1  POutMin=[]  POutMax=[]  IOutMin=[]  IOutMax=[]  DOutMin=[]  DOutMax=[]  NOutMin=[]  NOutMax=[]  SumOutMin=[]  SumOutMax=[]  SaturationOutMin=[]  SaturationOutMax=[]  PParamMin=[]  PParamMax=[]  IParamMin=[]  IParamMax=[]  DParamMin=[]  DParamMax=[]  NParamMin=[]  NParamMax=[]  KbParamMin=[]  KbParamMax=[]  KtParamMin=[]  KtParamMax=[]  KbOutMin=[]  KbOutMax=[]  KtOutMin=[]  KtOutMax=[]  IntegratorOutMin=[]  IntegratorOutMax=[]  FilterOutMin=[]  FilterOutMax=[]  SumI1OutMin=[]  SumI1OutMax=[]  SumI2OutMin=[]  SumI2OutMax=[]  SumI3OutMin=[]  SumI3OutMax=[]  SumI4OutMin=[]  SumI4OutMax=[]  SumDOutMin=[]  SumDOutMax=[]  DifferentiatorOutMin=[]  DifferentiatorOutMax=[]  FilterDiffOutCoefMin=[]  FilterDiffOutCoefMax=[]  ReciprocalOutMin=[]  ReciprocalOutMax=[]  SumDenOutMin=[]  SumDenOutMax=[]  SumNumOutMin=[]  SumNumOutMax=[]  DivideOutMin=[]  DivideOutMax=[]  UdiffTsProdOutMin=[]  UdiffTsProdOutMax=[]  NTsProdOutMin=[]  NTsProdOutMax=[]  UintegralTsProdOutMin=[]  UintegralTsProdOutMax=[]  UngainTsProdOutMin=[]  UngainTsProdOutMax=[]  IntegratorContinuousStateAttributes=''  IntegratorStateMustResolveToSignalObject=off  IntegratorRTWStateStorageClass=Auto  FilterContinuousStateAttributes=''  FilterStateMustResolveToSignalObject=off  FilterRTWStateStorageClass=Auto  ParallelPVariant=InternalParameters  IdealPVariant=Disabled  IVariant=InternalParameters  DVariant=Disabled  IntegratorVariant=Discrete  SatVariant=Disabled  AWVariant=Passthrough  PCopyVariant=Disabled  TRVariant=Disabled  FdbkBlocksVariant=Forward  IdealPFdbkVariant=Disabled  SatFdbkVariant=Disabled  DerivativeFilterVariant=Disabled  NVariant=Disabled  NCopyVariant=Disabled_SignalSpec  FilterICVariant=Disabled  IntegratorICVariant=InternalICs  ExternalResetVariant=Disabled  TRSumVariant=Passthrough  SumFdbkVariant=Disabled  SumVariant=Sum_PI  TsampFilterVariant=InternalTs  TsampNgainVariant=Passthrough  TsampIntegralVariant=Passthrough  ExternalSaturationOutDataTypeStr=Inherit: Same as second input
  PID Controller7 : slpidlib/PID Controller  Controller=PI  Form=Parallel  TimeDomain=Discrete-time  UseExternalTs=off  SampleTime=Ts  IntegratorMethod=Forward Euler  FilterMethod=Forward Euler  ControllerParametersSource=internal  P=50  I=0  D=0  UseFilter=on  N=100  TunerSelectOption=Transfer Function Based (PID Tuner App)  InitialConditionSource=internal  InitialConditionForIntegrator=0  InitialConditionForFilter=0  DifferentiatorICPrevScaledInput=0  ExternalReset=none  TrackingMode=off  Kt=1  LimitOutput=off  SatLimitsSource=internal  UpperSaturationLimit=inf  LowerSaturationLimit=-inf  LinearizeAsGain=on  AntiWindupMode=none  Kb=1  POutMin=[]  POutMax=[]  IOutMin=[]  IOutMax=[]  DOutMin=[]  DOutMax=[]  NOutMin=[]  NOutMax=[]  SumOutMin=[]  SumOutMax=[]  SaturationOutMin=[]  SaturationOutMax=[]  PParamMin=[]  PParamMax=[]  IParamMin=[]  IParamMax=[]  DParamMin=[]  DParamMax=[]  NParamMin=[]  NParamMax=[]  KbParamMin=[]  KbParamMax=[]  KtParamMin=[]  KtParamMax=[]  KbOutMin=[]  KbOutMax=[]  KtOutMin=[]  KtOutMax=[]  IntegratorOutMin=[]  IntegratorOutMax=[]  FilterOutMin=[]  FilterOutMax=[]  SumI1OutMin=[]  SumI1OutMax=[]  SumI2OutMin=[]  SumI2OutMax=[]  SumI3OutMin=[]  SumI3OutMax=[]  SumI4OutMin=[]  SumI4OutMax=[]  SumDOutMin=[]  SumDOutMax=[]  DifferentiatorOutMin=[]  DifferentiatorOutMax=[]  FilterDiffOutCoefMin=[]  FilterDiffOutCoefMax=[]  ReciprocalOutMin=[]  ReciprocalOutMax=[]  SumDenOutMin=[]  SumDenOutMax=[]  SumNumOutMin=[]  SumNumOutMax=[]  DivideOutMin=[]  DivideOutMax=[]  UdiffTsProdOutMin=[]  UdiffTsProdOutMax=[]  NTsProdOutMin=[]  NTsProdOutMax=[]  UintegralTsProdOutMin=[]  UintegralTsProdOutMax=[]  UngainTsProdOutMin=[]  UngainTsProdOutMax=[]  IntegratorContinuousStateAttributes=''  IntegratorStateMustResolveToSignalObject=off  IntegratorRTWStateStorageClass=Auto  FilterContinuousStateAttributes=''  FilterStateMustResolveToSignalObject=off  FilterRTWStateStorageClass=Auto  ParallelPVariant=InternalParameters  IdealPVariant=Disabled  IVariant=InternalParameters  DVariant=Disabled  IntegratorVariant=Discrete  SatVariant=Disabled  AWVariant=Passthrough  PCopyVariant=Disabled  TRVariant=Disabled  FdbkBlocksVariant=Forward  IdealPFdbkVariant=Disabled  SatFdbkVariant=Disabled  DerivativeFilterVariant=Disabled  NVariant=Disabled  NCopyVariant=Disabled_SignalSpec  FilterICVariant=Disabled  IntegratorICVariant=InternalICs  ExternalResetVariant=Disabled  TRSumVariant=Passthrough  SumFdbkVariant=Disabled  SumVariant=Sum_PI  TsampFilterVariant=InternalTs  TsampNgainVariant=Passthrough  TsampIntegralVariant=Passthrough  ExternalSaturationOutDataTypeStr=Inherit: Same as second input
  Product{,1..5} (6 alike) : Product
  Relational Operator : RelationalOperator  OutDataTypeStr=boolean  RndMeth=Simplest
  Relational Operator1 : RelationalOperator  OutDataTypeStr=boolean  RndMeth=Simplest
  Relational Operator2 : RelationalOperator  OutDataTypeStr=boolean  RndMeth=Simplest
  Scope{1..2,9..12,14..16} (9 alike) : Scope  NumInputPorts=3
  Scope13 : Scope  NumInputPorts=2
  Scope{3..4,6..7} (4 alike) : Scope  NumInputPorts=4
  Scope5 : Scope  NumInputPorts=6
  Scope8 : Scope  NumInputPorts=6
  Subsystem1 : Subsystem
      settings: PortSchema="{\"entries\":[{\"content\":{\"sides\":[{\"content\":{\"connectorIds\":[\"In1\",\"In2\",\"In3\"]},\"type\":\"ConnectorPlacement.EquallySpacedRectSide\",\"uuid\":\"61c1b8d0-ee8a-4339-8829-78338e22af7d\"},{\"content\":{\"connectorIds\":[\"Out1\",\"Out2\",\"Out3\",\"Out4\",\"Out5\",\"Out6\"],\"side\":\"RIGHT\"},\"type\":\"ConnectorPlacement.EquallySpacedRectSide\",\"uuid\":\"67da4172-786b-400a-a8d1-3fc67125f07d\"},{\"content\":{\"connectorIds\":[\"In4\"],\"side\":\"TOP\"},\"type\":\"ConnectorPlacement.EquallySpacedRectSide\",\"uuid\":\"4f4cbe20-6bcc-4d32-8788-836bef4ef16a\"}]},\"type\":\"ConnectorPlacement.EquallySpacedConnector\",\"uuid\":\"8ab0a139-c20a-4d51-a83b-5ca78b12ffd7\"}],\"packageUris\":[\"http://schema.mathworks.com/mf0/Connector/R2020b\"],\"version\":\"1.0\"}"
  Subsystem4 : Subsystem
  Sum{1..2,4..5,7..9,11,14..16} (11 alike) : Sum  Inputs=|+-
  Sum{3,6,10,12..13} (5 alike) : Sum  Inputs=|++
  Switch : Switch  Criteria=u2 > Threshold
  Triangle Generator : powerlib_meascontrol/Pulse & Signal Generators/Triangle Generator  Freq=10e3  Phase=90  Ts=0
  abc to dq2 : powerlib_meascontrol/Transformations/abc to dq0  Alignment=90 degrees behind phase A axis
  dq0 to abc : powerlib_meascontrol/Transformations/dq0 to abc  Alignment=90 degrees behind phase A axis
  dq0 to abc1 : powerlib_meascontrol/Transformations/dq0 to abc  Alignment=90 degrees behind phase A axis
  Pulse : Outport
  Id : Outport  Port=2
  wt_1 : Outport  Port=3
  wires:
  [Iq] -> Gain7/1
  [Id] -> Gain1/1
  [Id] -> Sum1/2, Scope7/2
  Enable/1 -> Product1/2, Product/2, Logical Operator7/2, Logical Operator3/2, Logical Operator4/2, Logical Operator5/2, Logical Operator8/2, Logical Operator6/2, Product3/2, Product2/2, Product4/2, Product5/2
  Product5/1 -> PID Controller6/1
  Sum16/1 -> Scope8/5, Product5/1
  Product4/1 -> PID Controller5/1
  Sum14/1 -> Product4/1
  Product3/1 -> PID Controller3/1
  Sum7/1 -> Product3/1, Scope4/3
  Product2/1 -> PID Controller4/1
  Sum11/1 -> Scope2/2, Product2/1
  Constant1/1 -> Scope6/1, Sum4/1
  Current/1 -> Sum1/1, Scope7/1
  dq0 to abc1/1 -> Scope10/3, Switch/3
  dq0 to abc/1 -> Scope9/3, Switch/1
  [Vd] -> Sum7/2, Scope4/2
  Sum8/1 -> Sum9/1, Scope5/2
  Constant2/1 -> Sum11/1
  [IqL] -> Sum12/2, Scope8/1
  PID Controller3/1 -> Sum8/1, Scope4/4
  Sum15/1 -> Mux1/1
  Gain7/1 -> Sum15/2
  Mux1/1 -> dq0 to abc1/1, Scope10/1
  Sum12/1 -> Sum13/1, Scope8/2
  PID Controller5/1 -> Scope5/6, Sum15/1
  PID Controller6/1 -> Scope8/6, Sum10/1
  [Id] -> Gain8/1
  Gain5/1 -> Sum9/2
  Gain6/1 -> Sum13/2, Scope8/3
  PID Controller4/1 -> Scope2/3, Sum12/1
  Gain8/1 -> Sum10/2
  Sum13/1 -> Sum16/1, Scope8/4
  [Vq] -> Gain5/1
  Sum10/1 -> Mux1/2
  [wt] -> dq0 to abc/2, Scope9/2, Scope10/2, dq0 to abc1/2
  [Vq] -> Scope2/1, Sum11/2
  Sum9/1 -> Sum14/1, Scope5/4
  [Vd] -> Gain6/1
  Constant3/1 -> Sum7/1, Scope4/1
  mode/1 -> [breaker], Switch/2
  Product1/1 -> PID Controller1/1
  [Iq] -> Gain/1, Scope6/2, Sum4/2
  Gain1/1 -> Sum5/2
  Sum4/1 -> Scope6/3, Product/1
  Sum2/1 -> Sum3/1, Scope11/1
  Sum5/1 -> Sum6/1, Scope12/1
  PID Controller2/1 -> Scope6/4, Sum5/1
  Mux/1 -> dq0 to abc/1, Scope9/1
  Sum1/1 -> Scope7/3, Product1/1
  Sum3/1 -> Scope11/3, Mux/1
  [Vq] -> Sum6/2, Scope12/2
  Sum6/1 -> Scope12/3, Mux/2
  Product/1 -> PID Controller2/1
  Gain/1 -> Sum2/2
  [Vd] -> Sum3/2, Scope11/2
  PID Controller1/1 -> Sum2/1, Scope7/4
  Divide2/1 -> Relational Operator2/1
  Gain4/1 -> Divide2/1
  Gain3/1 -> Divide1/1
  Divide1/1 -> Relational Operator1/1
  Vbus1/1 -> Divide/2, Divide1/2, Divide2/2
  Divide/1 -> Relational Operator/1, Scope3/2
  Gain2/1 -> Divide/1
  Logical Operator8/1 -> Bus Creator/1
  Logical Operator7/1 -> Bus Creator/2
  Logical Operator6/1 -> Bus Creator/3
  Logical Operator5/1 -> Bus Creator/4
  Logical Operator1/1 -> Logical Operator5/1
  Logical Operator4/1 -> Bus Creator/5
  Logical Operator2/1 -> Logical Operator3/1
  Logical Operator3/1 -> Bus Creator/6
  Bus Creator/1 -> Pulse/1
  Logical Operator/1 -> Logical Operator7/1, Scope3/4
  Demux3/1 -> Gain2/1
  Relational Operator/1 -> Logical Operator/1, Scope3/3, Logical Operator8/1
  Triangle Generator/1 -> Scope3/1, Relational Operator/2, Relational Operator1/2, Relational Operator2/2
  Relational Operator1/1 -> Logical Operator1/1, Logical Operator6/1
  Relational Operator2/1 -> Logical Operator2/1, Logical Operator4/1
  Switch/1 -> Demux3/1
  Demux3/3 -> Gain4/1
  Demux3/2 -> Gain3/1
  [Vd] -> Subsystem4/1(Vd)
  [Iq] -> Subsystem4/4(Iq)
  Iabc/1 -> Subsystem1/2(Iabc)
  Demux2/1 -> [IdL], Scope14/1
  Demux2/2 -> [IqL], Scope14/2
  Subsystem1/5(Iq) -> [Iq], Scope16/2
  abc to dq2/1 -> Demux2/1
  [wt] -> abc to dq2/2
  Subsystem4/2(REACTIVA) -> Scope15/2
  [wt] -> Subsystem1/3(w)
  Subsystem1/3(dq0) -> Scope1/3
  Subsystem4/1(ACTIVA) -> Scope15/1
  Iabcl1/1 -> abc to dq2/1, Scope13/2
  [Id] -> Subsystem4/3(Id)
  Subsystem1/1(Vd) -> [Vd], Scope1/1
  [breaker] -> Subsystem1/4(breaker)
  Subsystem4/3(APARENTE) -> Scope15/3
  [Vq] -> Subsystem4/2(Vq)
  Subsystem1/6(wt) -> Scope16/3, wt_1/1, [wt]
  Vabc/1 -> Subsystem1/1(Vabc), Scope13/1
  Subsystem1/2(Vq) -> [Vq], Scope1/2
  Subsystem1/4(Id) -> Scope16/1, Id/1, [Id]
  Demux2/3 -> Scope14/3
  [Iq] -> Sum16/2
  Constant5/1 -> Sum8/2
  Constant4/1 -> Sum14/2
